simulink model "LQR_model"  (R2021a)
settings: Solver=VariableStepAuto  StartTime=0.0  StopTime=10  MaxStep=1e-4  RelTol=1e-9
values from neighbouring files (symbols this model uses):
  A = [0 -(1-D_ss)/L; (1-D_ss)/C -1/(R*C)]    [tranfer_func_ex4.m]
  B = [Vo_ss/L; -iL_ss/C]    [tranfer_func_ex4.m]
undefined symbols (not defined in the file or in its folder): K_LQ
settings Model: Creator=panos  LastModifiedBy=nikol
settings DebuggingCC: UnconnectedInputMsg=none  UnconnectedOutputMsg=none  UnconnectedLineMsg=none
settings ModelReferenceCC: EnableRefExpFcnMdlSchedulingChecks=off
settings RTWCC: Description=Generic Real-Time Target  DLArmComputeVersion=20.02.1

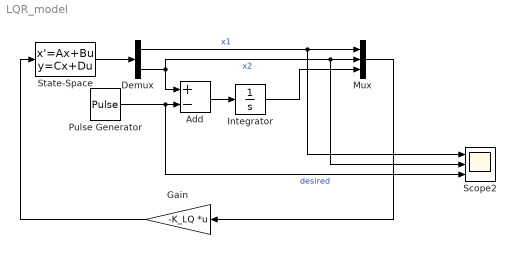
== system LQR_model ==
  Add : Sum  Inputs=+-
  Demux : Demux  Outputs=2
  Gain : Gain  Gain=-K_LQ  Multiplication=Matrix(K*u)
  Integrator : Integrator
  Mux : Mux  Inputs=3
  Pulse Generator : DiscretePulseGenerator  PulseType=Time based  Period=3  PulseWidth=30
  Scope2 : Scope  NumInputPorts=3
  State-Space : StateSpace  A=A  B=B  C=eye(2)  D=[0;0]  InitialCondition=[2,0]
  wires:
  State-Space/1 -> Demux/1
  Mux/1 -> Gain/1
  Gain/1 -> State-Space/1
  Demux/1 -> Mux/1, Scope2/1  "x1"
  Demux/2 -> Add/1, Scope2/2, Mux/2  "x2"
  Integrator/1 -> Mux/3
  Pulse Generator/1 -> Scope2/3, Add/2  "desired"
  Add/1 -> Integrator/1
